simulink model "first"  (R2024a)
settings: Solver=FixedStepAuto  StartTime=0.0  StopTime=5  FixedStep=0.0001  RelTol=1e-3
values from neighbouring files (symbols this model uses):
  k1 = (1 - z1)/(K_CO*T)    (= 1.73611111111)    [first_calc.m]
  k2 = (1 - z2)/(K_CO*T)    (= 1.38888888889)    [first_calc.m]
  k3 = (1 - z3)/(K_CO*T)    (= 1.04166666667)    [first_calc.m]
  k4 = (1 - z4)/(K_CO*T)    (= 0.694444444444)    [first_calc.m]
  k5 = (1 - z5)/(K_CO*T)    (= 0.347222222222)    [first_calc.m]
  k6 = (1 - z6)/(K_CO*T)    (= 0)    [first_calc.m]
  k7 = (1 - z7)/(K_CO*T)    (= -0.347222222222)    [first_calc.m]
  K_CO = 7.2    [first_calc.m]
  K_FB = 1    [first_calc.m]
  T = 0.2    [first_calc.m]
settings Model: Creator=ventus  LastModifiedBy=ventus

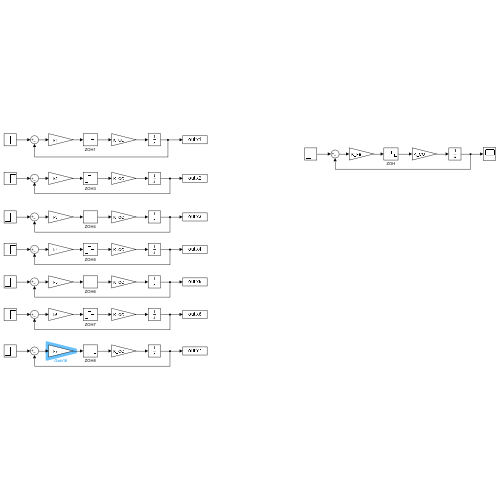
[thumbnail: Simulink's stored preview of the top-level diagram]
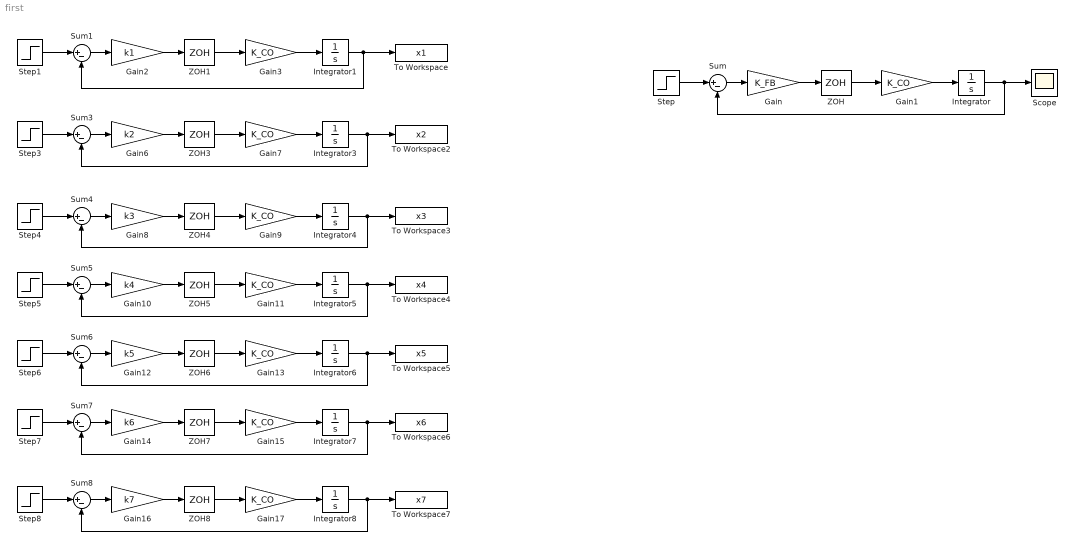
== system first ==
  Gain : Gain  Gain=K_FB
  Gain{1,3,7,9,11,13,15,17} (8 alike) : Gain  Gain=K_CO
  Gain10 : Gain  Gain=k4
  Gain12 : Gain  Gain=k5
  Gain14 : Gain  Gain=k6
  Gain16 : Gain  Gain=k7
  Gain2 : Gain  Gain=k1
  Gain6 : Gain  Gain=k2
  Gain8 : Gain  Gain=k3
  Integrator{,1,3..8} (8 alike) : Integrator
  Scope : Scope
  Step{,1,3..8} (8 alike) : Step  SampleTime=0
  Sum{,1,3..8} (8 alike) : Sum  Inputs=|+-
  To Workspace : ToWorkspace  VariableName=x1  SaveFormat=Timeseries  SampleTime=-1
  To Workspace2 : ToWorkspace  VariableName=x2  SaveFormat=Timeseries  SampleTime=-1
  To Workspace3 : ToWorkspace  VariableName=x3  SaveFormat=Timeseries  SampleTime=-1
  To Workspace4 : ToWorkspace  VariableName=x4  SaveFormat=Timeseries  SampleTime=-1
  To Workspace5 : ToWorkspace  VariableName=x5  SaveFormat=Timeseries  SampleTime=-1
  To Workspace6 : ToWorkspace  VariableName=x6  SaveFormat=Timeseries  SampleTime=-1
  To Workspace7 : ToWorkspace  VariableName=x7  SaveFormat=Timeseries  SampleTime=-1
  ZOH{,1,3..8} (8 alike) : ZeroOrderHold  SampleTime=T
  wires:
  Step/1 -> Sum/1
  Sum/1 -> Gain/1
  Gain/1 -> ZOH/1
  ZOH/1 -> Gain1/1
  Gain1/1 -> Integrator/1
  Integrator/1 -> Sum/2, Scope/1
  ZOH1/1 -> Gain3/1
  Sum1/1 -> Gain2/1
  Integrator1/1 -> To Workspace/1, Sum1/2
  Gain3/1 -> Integrator1/1
  Gain2/1 -> ZOH1/1
  Step1/1 -> Sum1/1
  Gain7/1 -> Integrator3/1
  Step3/1 -> Sum3/1
  Integrator3/1 -> To Workspace2/1, Sum3/2
  Gain6/1 -> ZOH3/1
  ZOH3/1 -> Gain7/1
  Sum3/1 -> Gain6/1
  Gain9/1 -> Integrator4/1
  Step4/1 -> Sum4/1
  Integrator4/1 -> To Workspace3/1, Sum4/2
  Gain8/1 -> ZOH4/1
  ZOH4/1 -> Gain9/1
  Sum4/1 -> Gain8/1
  Gain11/1 -> Integrator5/1
  Step5/1 -> Sum5/1
  Integrator5/1 -> To Workspace4/1, Sum5/2
  Gain10/1 -> ZOH5/1
  ZOH5/1 -> Gain11/1
  Sum5/1 -> Gain10/1
  Gain13/1 -> Integrator6/1
  Step6/1 -> Sum6/1
  Integrator6/1 -> To Workspace5/1, Sum6/2
  Gain12/1 -> ZOH6/1
  ZOH6/1 -> Gain13/1
  Sum6/1 -> Gain12/1
  Gain15/1 -> Integrator7/1
  Step7/1 -> Sum7/1
  Integrator7/1 -> To Workspace6/1, Sum7/2
  Gain14/1 -> ZOH7/1
  ZOH7/1 -> Gain15/1
  Sum7/1 -> Gain14/1
  Gain17/1 -> Integrator8/1
  Step8/1 -> Sum8/1
  Integrator8/1 -> To Workspace7/1, Sum8/2
  Gain16/1 -> ZOH8/1
  ZOH8/1 -> Gain17/1
  Sum8/1 -> Gain16/1
